simulink model "AttitudeEstimation"  (Simulink 9.1)
settings: Solver=FixedStepDiscrete  StartTime=startTime  StopTime=stopTime  FixedStep=TA  RelTol=1e-3
settings Model: SuppressorTable=22 serialization::archive 11 0 6 0 0 0 1 0  Creator=martin  LastModifiedBy=martin
settings DataIOCC: SaveFormat=Dataset
settings OptimizationCC: EnhancedBackFolding=on  PassReuseOutputArgsAs=Individual arguments  ZeroExternalMemoryAtStartup=off  ZeroInternalMemoryAtStartup=off  InitFltsAndDblsToZero=on  EfficientMapNaN2IntZero=off  LifeSpan=auto  BufferReusableBoundary=off  OptimizeBlockOrder=speed  DifferentSizesBufferReuse=on  OptimizationCustomize=off
settings DebuggingCC: UnderspecifiedInitializationDetection=Simplified  MergeDetectMultiDrivingBlocksExec=error  ParameterTunabilityLossMsg=error  BusObjectLabelMismatch=error  SFUnexpectedBacktrackingDiag=error  SFNoUnconditionalDefaultTransitionDiag=error  SFExecutionAtInitializationDiag=warning
settings HardwareCC: ProdBitPerPointer=64  ProdBitPerSizeT=64  ProdBitPerPtrDiffT=64  ProdLargestAtomicFloat=Float  ProdIntDivRoundTo=Zero  ProdEndianess=LittleEndian  ProdWordSize=64  ProdHWDeviceType=Intel->x86-64 (Windows64)
settings ModelReferenceCC: PropagateSignalLabelsOutOfModel=on
settings SFSimCC: MATLABDynamicMemAlloc=off
settings RTWCC: SystemTargetFile=ert.tlc  GenCodeOnly=on  PackageGeneratedCodeAndArtifacts=on  TemplateMakefile=ert_default_tmf  Description=Embedded Coder  GenerateReport=on  IncludeHyperlinkInReport=on  LaunchReport=on  TargetLang=C++  GenerateTraceInfo=on  GenerateTraceReport=on  GenerateTraceReportSl=on  GenerateTraceReportSf=on  GenerateTraceReportEml=on
settings CodeAppCC: ForceParamTrailComments=on  IgnoreCustomStorageClasses=off  OperatorAnnotations=on  SimulinkDataObjDesc=on  SFDataObjDesc=on  InsertBlockDesc=on  StateflowObjectComments=off
settings ERTTargetCC: TargetLangStandard=C++03 (ISO)  GenerateSampleERTMain=on  MultiInstanceERTCode=on  CodeInterfacePackaging=C++ class  MultiInstanceErrorCode=Warning  RootIOFormat=Structure reference  ERTCustomFileTemplate=example_file_process.tlc
settings CPPComponent: GenerateDestructor=on  GenerateExternalIOAccessMethods=Structure-based method  ParameterMemberVisibility=private  InternalMemberVisibility=private  GenerateParameterAccessMethods=Method  GenerateInternalMemberAccessMethods=None  UseOperatorNewForModelRefRegistration=off
settings ConfigComp: CovMetricSettings=dwe  CovHtmlReporting=off  CovSaveCumulativeToWorkspaceVar=off  CovSaveSingleToWorkspaceVar=off  CovExternalEMLEnable=on

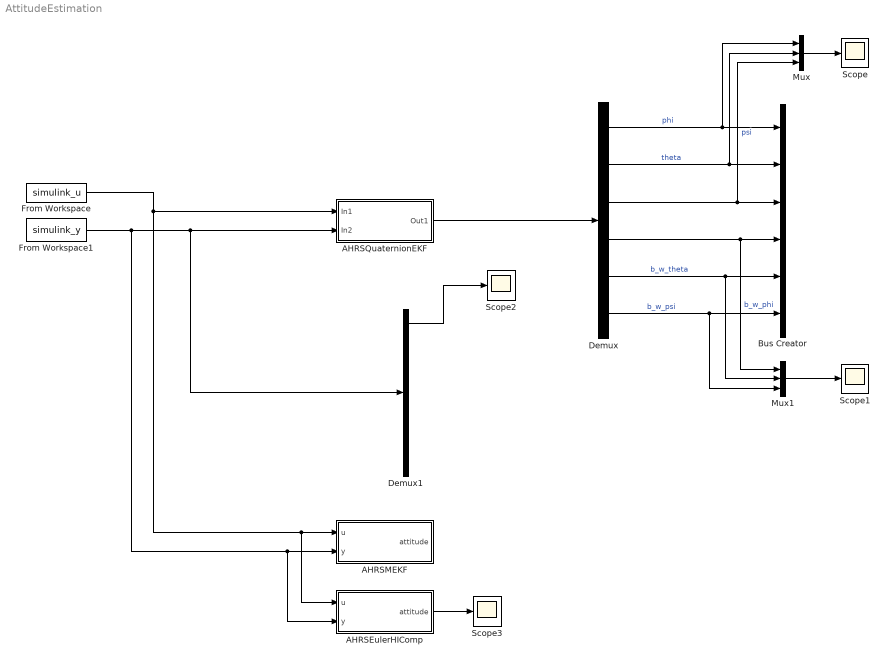
== system AttitudeEstimation ==
  AHRSEulerHIComp : Subsystem  TreatAsAtomicUnit=on
  AHRSMEKF : Subsystem  TreatAsAtomicUnit=on
  AHRSQuaternionEKF : Subsystem  TreatAsAtomicUnit=on
  Bus Creator : BusCreator  Inputs=6
  Demux : Demux  Outputs=6
  Demux1 : Demux  Outputs=6
  From Workspace : FromWorkspace  VariableName=simulink_u  SampleTime=0
  From Workspace1 : FromWorkspace  VariableName=simulink_y  SampleTime=0
  Mux : Mux  Inputs=3
  Mux1 : Mux  Inputs=3
  Scope{,1..3} (4 alike) : Scope
  wires:
  From Workspace/1 -> AHRSEulerHIComp/1(u), AHRSMEKF/1(u), AHRSQuaternionEKF/1(In1)
  From Workspace1/1 -> AHRSEulerHIComp/2(y), AHRSMEKF/2(y), Demux1/1, AHRSQuaternionEKF/2(In2)
  AHRSQuaternionEKF/1(Out1) -> Demux/1
  Demux/1 -> Mux/1, Bus Creator/1  "phi"
  Demux/2 -> Mux/2, Bus Creator/2  "theta"
  Demux/3 -> Mux/3, Bus Creator/3  "psi"
  Demux/4 -> Mux1/1, Bus Creator/4  "b_w_phi"
  Demux/5 -> Mux1/2, Bus Creator/5  "b_w_theta"
  Demux/6 -> Mux1/3, Bus Creator/6  "b_w_psi"
  Mux/1 -> Scope/1
  Mux1/1 -> Scope1/1
  Demux1/1 -> Scope2/1
  AHRSEulerHIComp/1(attitude) -> Scope3/1

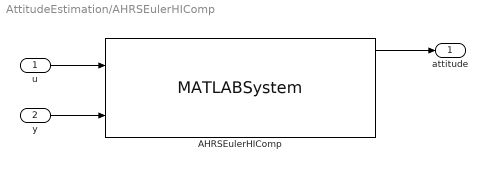
== system AttitudeEstimation/AHRSEulerHIComp ==
  u : Inport
  y : Inport  Port=2
  AHRSEulerHIComp : MATLABSystem  System=AHRSEulerEKFHIComp  sampleTime=TA  delta_i=delta_i  delta_d=delta_d  g_mps2=g_mps2  x0=x0_eulerEKFHIComp  P0=P0_eulerEKFHIComp  sigma_2_w=sigma2.w_b  sigma_2_a=sigma2.a_b  sigma_2_b_w=sigma2.b_w  sigma_2_yaw=sigma2.mag  SimulateUsing=Interpreted execution
      mask Type: AHRSEulerEKFHIComp
      mask Display:
      | disp('AHRSEulerEKFHIComp');
      | port_label('input',1,'u');
      | port_label('input',2,'y');
      | port_label('output',1,'attitude');
      | port_label('output',2,'b_w');
      | port_label('output',3,'m_e');
      | port_label('output',4,'m_b');
  attitude : Outport
  wires:
  u/1 -> AHRSEulerHIComp/1
  y/1 -> AHRSEulerHIComp/2
  AHRSEulerHIComp/1 -> attitude/1

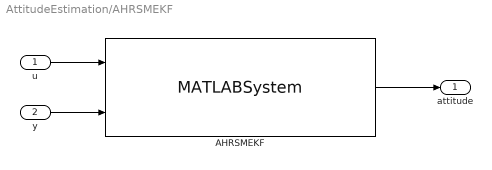
== system AttitudeEstimation/AHRSMEKF ==
  u : Inport
  y : Inport  Port=2
  AHRSMEKF : MATLABSystem  System=AHRSMEKF  sigma_2_w=sigma2.w_b  sigma_2_a=sigma2.a_b  sigma_2_b_w=sigma2.b_w  sigma_2_yaw=sigma2.mag  sampleTime=TA  delta_i=delta_i  delta_d=delta_d  g_mps2=g_mps2  SimulateUsing=Code generation
      mask Type: AHRSMEKF
      mask Display:
      | disp('AHRSMEKF');
      | port_label('input',1,'u');
      | port_label('input',2,'y');
      | port_label('output',1,'attitude');
  attitude : Outport
  wires:
  u/1 -> AHRSMEKF/1
  y/1 -> AHRSMEKF/2
  AHRSMEKF/1 -> attitude/1

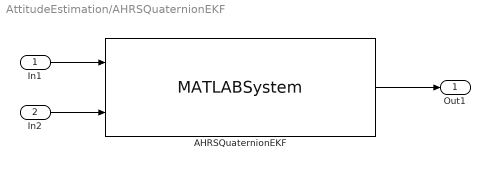
== system AttitudeEstimation/AHRSQuaternionEKF ==
  In1 : Inport
  In2 : Inport  Port=2
  AHRSQuaternionEKF : MATLABSystem  System=AHRSQuaternionEKF  sigma_2_quaternion=sigma2.quaternion  sigma_2_b_w=sigma2.b_w  sigma_2_a=sigma2.a_b  sigma_2_yaw=sigma2.mag  TA=TA  delta_i=delta_i  delta_d=delta_d  g_mps2=g_mps2  P0=P0_quaternionEKF  x0=x0_quaternionEKF  SimulateUsing=Interpreted execution
      mask Type: AHRSQuaternionEKF
      mask Display:
      | disp('AHRSQuaternionEKF');
      | port_label('input',1,'u');
      | port_label('input',2,'y');
      | port_label('output',1,'states');
  Out1 : Outport
  wires:
  In1/1 -> AHRSQuaternionEKF/1
  In2/1 -> AHRSQuaternionEKF/2
  AHRSQuaternionEKF/1 -> Out1/1
